simulink library "VACLib"  (R2022b)
settings: Solver=VariableStepAuto  StartTime=0.0  StopTime=10.0  RelTol=1e-3
settings Model: Creator=KarlO  LastModifiedBy=KarlO

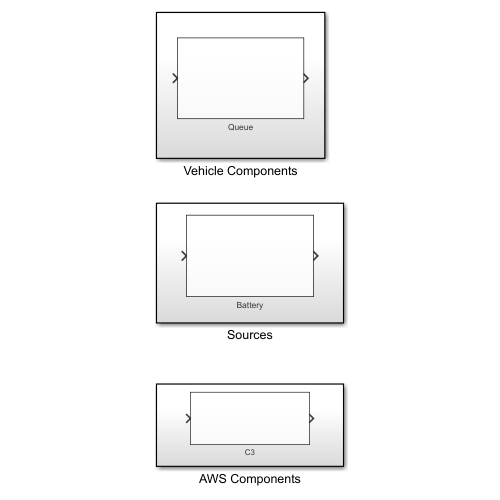
[thumbnail: Simulink's stored preview of the top-level diagram]
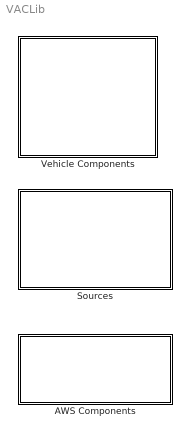
== system VACLib ==
  AWS Components : Subsystem
  Sources : Subsystem
  Vehicle Components : Subsystem

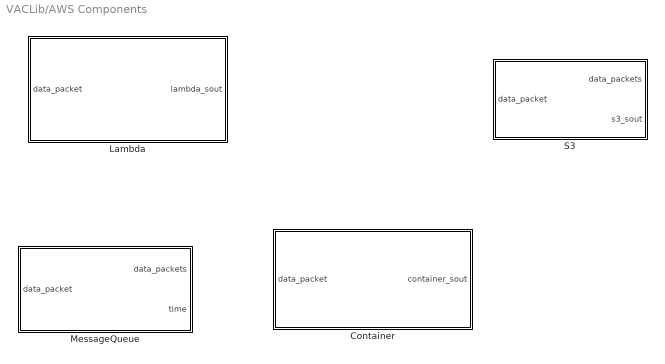
== system VACLib/AWS Components ==
  Container : MATLAB Function  TreatAsAtomicUnit=on  mask{no_cores=1, ram=8, no_instances=1}
      mask prompts: no_cores "Number of Cores"; no_instances "Number of Instances"
  Lambda : MATLAB Function  TreatAsAtomicUnit=on  mask{no_instances=1}
      mask prompts: no_instances "Number of Instances"
  MessageQueue : MATLAB Function  TreatAsAtomicUnit=on  mask{queue_size=32}
      mask prompts: queue_size "Queue Size"
  S3 : MATLAB Function  TreatAsAtomicUnit=on  mask{consistency=0}

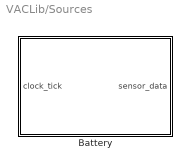
== system VACLib/Sources ==
  Battery : MATLAB Function  TreatAsAtomicUnit=on  mask{sensor_data_size=8}
      mask prompts: sensor_data_size "Sensor Data Size (kB)"

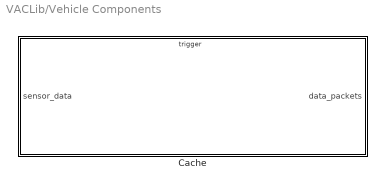
== system VACLib/Vehicle Components ==
  Cache : MATLAB Function  TreatAsAtomicUnit=on  mask{cache_size=32}
      mask prompts: cache_size "Cache Size"

== matlab function VACLib/Vehicle Components/Cache ==
  data: sensor_data input double; data_packets output double; cache_size parameter
  events: trigger input EITHER_EDGE_EVENT
function data_packets = cache(sensor_data, cache_size)
%Start timer
tic;
persistent accumulated_data;
if isempty(accumulated_data)
    accumulated_data = 0;
end

%Set time since packet last sent
time_since_last_send = toc;

accumulated_data = accumulated_data + sensor_data;
if accumulated_data >= cache_size || time_since_last_send >= 5
    data_packets = accumulated_data;
    accumulated_data = 0;
    tic;
else
    data_packets = 0;
end

== matlab function VACLib/AWS Components/S3 ==
  data: data_packet input; data_packets output; consistency parameter; s3_sout output
function [data_packets, s3_sout] = S3(data_packet, consistency)
%Consistency should be 0, 1 or 2, and corresponds to different consistency
%types
persistent s3_time;
persistent s3_cost;

if isempty(s3_cost)
    s3_cost = 0;
end
if isempty(s3_time)
    s3_time = 0;
end

switch consistency
    case 1
        %Based on consistency type, divide into read units per cost
        data_packets = data_packet;
        delay_time = 10;
        s3_time = s3_time + delay_time;
        s3_cost = s3_cost + 10;
    case 2
        data_packets = data_packet;
        delay_time = 5;
        s3_time = s3_time + delay_time;
        s3_cost = s3_cost + 50;
    case 3
        data_packets = data_packet;
        delay_time = 1;
        s3_time = s3_time + delay_time;
        s3_cost = s3_cost + 100;
    otherwise
        error('Invalid consistency type');
end
s_time = s3_time;
s_cost = s3_cost;
s3_sout = [s_time, s_cost];
end

== matlab function VACLib/Sources/Battery ==
  data: clock_tick input; sensor_data output; sensor_data_size parameter
function sensor_data = battery(clock_tick, sensor_data_size)

sensor_data = clock_tick * sensor_data_size;

== matlab function VACLib/AWS Components/Lambda ==
  data: data_packet input; lambda_sout output; no_instances parameter
function lambda_sout  = lambda(data_packet, no_instances)
%Price of lambda instance depends on memory allocated to it
%An increase in memory size triggers an equivalent increase in CPU available to your function.

%TODO - Add batching to cost model and paramter

persistent lambda_cost;
persistent lambda_time;
persistent total_requests;
persistent request_cost;

if isempty(total_requests)
    total_requests = 0;
end
if isempty(request_cost)
    request_cost = 0;
end
if isempty(lambda_time)
    lambda_time = 0;
end

if isempty(lambda_cost)
    lambda_cost = 0;
end


total_requests = total_requests + 1;

%Request cost for a AWS lambda resource to request the data from source
%(S3) per second
request_cost = request_cost + (total_requests * 0.0000002);

%Average compute duration in sec
avg_dur = 2;

%Memory allocated to each instance in MB
allocated_mem = 1024;

%Monthly compute duration in seconds -NEED TRIGGER TO ONLY RUN WHEN THERE
%ARE NO MORE SIGNALS
monthly_compute_dur = total_requests * avg_dur;

%Monthly compute GB-s
monthly_compute = monthly_compute_dur * (allocated_mem / 1024);

%Cost per second, to keep cost parameter consistent throughout system
cost_per_sec = monthly_compute / 2630000;

%Total cost for running a lambda instance for one second, multiplied by a
%factor based on the number of lambda instances initiated
lambda_cost = lambda_cost + ((cost_per_sec + request_cost)*(no_instances*0.5));

%Total time should be proportional throughout the system
lambda_time = lambda_time + 1;

lambda_sout = [lambda_time, lambda_cost];

== matlab function VACLib/AWS Components/Container ==
  data: data_packet input; no_cores parameter; container_sout output; no_instances parameter; ram parameter
function container_sout  = container(data_packet, no_cores, no_instances, ram)

persistent container_cost;
persistent container_time;

if isempty(container_time)
    container_time = 0;
end
if isempty(container_cost)
    container_cost = 0;
end

container_cost = container_cost + (no_cores*10) + (ram*2) + (no_instances*100);
container_time = container_time + data_packet/no_instances;

container_sout = [container_time, container_cost];

== matlab function VACLib/AWS Components/MessageQueue ==
  data: data_packet input; data_packets output; time output; queue_size parameter
function [data_packets, time] = messageQueue(data_packet, queue_size)
%Start timer
tic;
%For future reference. Message queue should send the buffered data at the
%end of simulation so that data does not get lost and messes up cost model.
persistent accumulated_data;
if isempty(accumulated_data)
    accumulated_data = 0;
end
%Set time since packet last sent
time_since_last_send = toc;

accumulated_data = accumulated_data + data_packet;
%Time threshold to wait if no data is receieved
if accumulated_data >= queue_size || time_since_last_send >= 5
    data_packets = accumulated_data;
    accumulated_data = 0;
    time = time_since_last_send;
    tic;
else
    data_packets = 0;
    time = 0;
end

%TODO - Få batteriet att skicka i 10 sec, simulationen att köra i 15.
